simulink model "Exp2_Observation_1_PCM"  (R2020b)
settings: Solver=VariableStepAuto  StartTime=0.0  StopTime=10.0  RelTol=1e-3
libraries: commutil2 x2, dspquant2 x2, dsparch4 x1, dspsigops x1
settings Model: Creator=Mohit Akhouri  LastModifiedBy=Mohit Akhouri

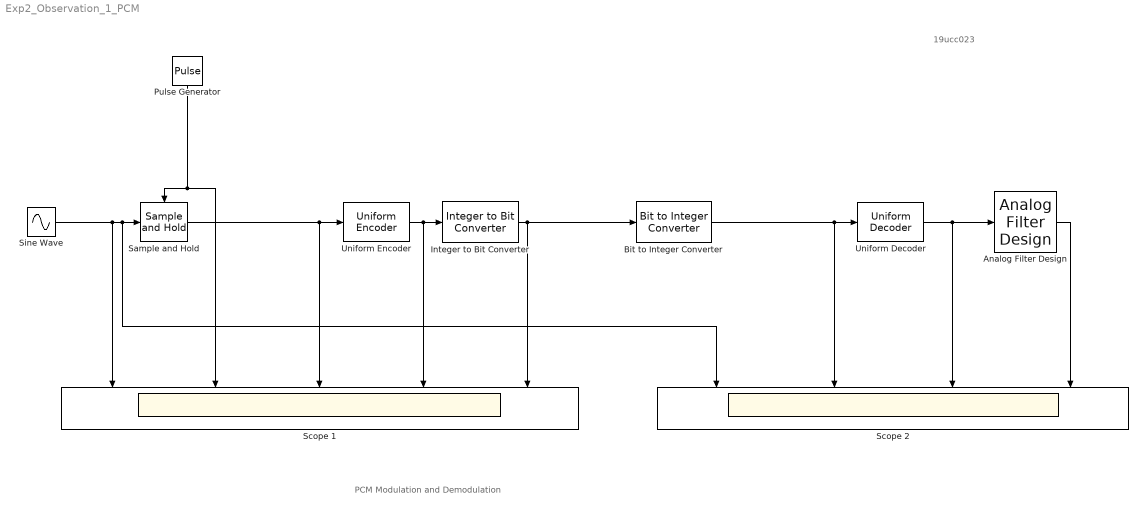
== system Exp2_Observation_1_PCM ==
  note: PCM Modulation and Demodulation
  note: 19ucc023
  Analog Filter Design : dsparch4/Analog Filter Design  method=Butterworth  filttype=Lowpass  N=8  Wlo=2*pi*2  Whi=80  Rp=2  Rs=40
  Bit to Integer Converter : commutil2/Bit to Integer Converter  nbits=4  bitOrder=MSB first  signedOutputValues=Unsigned  outDtype=Inherit via internal rule  outDtypeSigned=Inherit via internal rule
  Integer to Bit Converter : commutil2/Integer to Bit Converter  nbits=4  signedInputValues=Unsigned  bitOrder=MSB first  outDtype=Inherit via internal rule
  Pulse Generator : DiscretePulseGenerator  PulseType=Time based  Amplitude=5  Period=1/20  PulseWidth=50
  Sample and Hold : dspsigops/Sample and Hold  trig=Rising edge  initCond=0  latchinput=off
  Scope 1 : Scope  NumInputPorts=5
  Scope 2 : Scope  NumInputPorts=4
  Sine Wave : Sin  Amplitude=5  Frequency=2*pi*2  SampleTime=0
  Uniform Decoder : dspquant2/Uniform Decoder  peak=5  bits=4  overflowMode=Saturate  otype=Double
      settings: SourceProductBaseCode=DS
  Uniform Encoder : dspquant2/Uniform Encoder  peak=5  bits=4  otype=Unsigned integer
  wires:
  Pulse Generator/1 -> Scope 1/2, Sample and Hold/Trigger
  Sine Wave/1 -> Sample and Hold/1, Scope 2/1, Scope 1/1
  Sample and Hold/1 -> Scope 1/3, Uniform Encoder/1
  Uniform Encoder/1 -> Scope 1/4, Integer to Bit Converter/1
  Integer to Bit Converter/1 -> Bit to Integer Converter/1, Scope 1/5
  Bit to Integer Converter/1 -> Scope 2/2, Uniform Decoder/1
  Uniform Decoder/1 -> Scope 2/3, Analog Filter Design/1
  Analog Filter Design/1 -> Scope 2/4
